simulink model "smc_rotary_pendulam"  (R2023b)
settings: Solver=VariableStepAuto  StartTime=0.0  StopTime=20  RelTol=1e-3
values from neighbouring files (symbols this model uses):
  A = double(J_subs(:,1:4))    [smc_rotary_pendulam_setup.m]
  B = double(J_subs(:,5))    [smc_rotary_pendulam_setup.m]
  D = [0,0,0,0]    [smc_rotary_pendulam_setup.m]
  K_lin = lqr(A,B,Q_1,R_1)    [smc_rotary_pendulam_setup.m]
  K_nom = -(sliding_surface*A)    [smc_rotary_pendulam_setup.m]
  sliding_surface = transpose(eig_vec(:,2))/(transpose(eig_vec(:,2))*B)    [smc_rotary_pendulam_setup.m]
undefined symbols (not defined in the file or in its folder): eig_val
libraries: simulink_extras x6
settings Model: Creator=Harishankar  LastModifiedBy=Harishankar

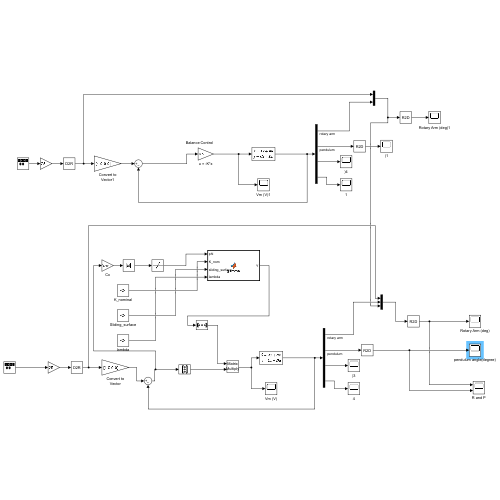
[thumbnail: Simulink's stored preview of the top-level diagram]
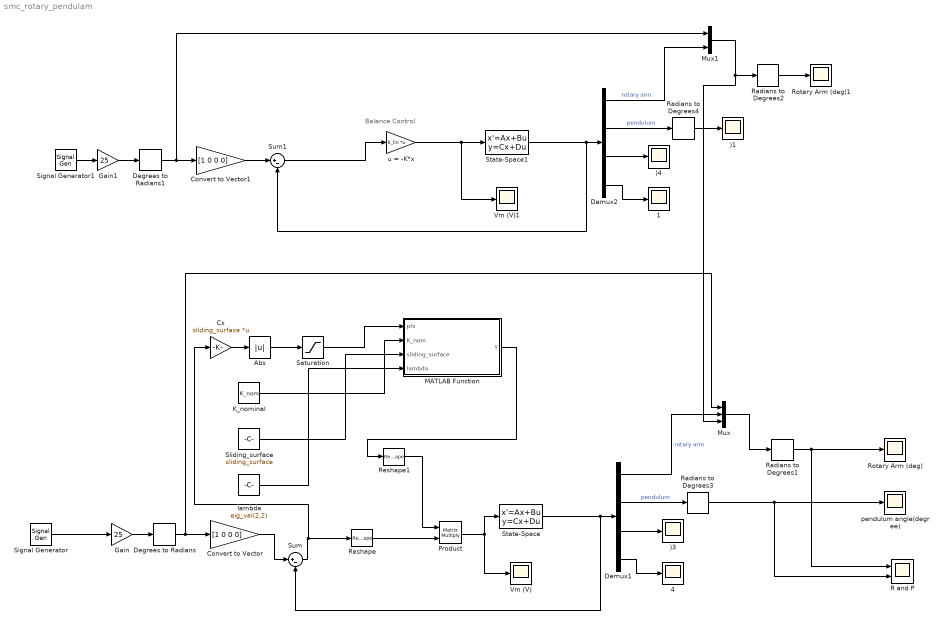
== system smc_rotary_pendulam ==
  note: Balance Control
  )1 : Scope
  )3 : Scope
  )4 : Scope
  1 : Scope
  4 : Scope
  Abs : Abs  SaturateOnIntegerOverflow=off
  Convert to Vector : Gain  Gain=[1 0 0 0]
  Convert to Vector1 : Gain  Gain=[1 0 0 0]
  Cx : Gain  Gain=sliding_surface  Multiplication=Matrix(K*u) (u vector)
  Degrees to Radians : simulink_extras/Transformations/Degrees to Radians
  Degrees to Radians1 : simulink_extras/Transformations/Degrees to Radians
  Demux1 : Demux
  Demux2 : Demux
  Gain : Gain  Gain=25
  Gain1 : Gain  Gain=25
  K_nominal : Constant  Value=K_nom
  MATLAB Function : MATLAB Function  TreatAsAtomicUnit=on
  Mux : Mux  Inputs=3
  Mux1 : Mux  Inputs=2
  Product : Product  Multiplication=Matrix(*)
  R and P : Scope  NumInputPorts=2
  Radians to Degrees{1..4} (4 alike) : simulink_extras/Transformations/Radians to Degrees
  Reshape : Reshape  OutputDimensionality=Column vector (2-D)
  Reshape1 : Reshape  OutputDimensionality=Row vector (2-D)
  Rotary Arm (deg) : Scope
  Rotary Arm (deg)1 : Scope
  Saturation : Saturate  UpperLimit=1  LowerLimit=0.35  LinearizeAsGain=off
  Signal Generator : SignalGenerator  WaveForm=square  Frequency=0.125
  Signal Generator1 : SignalGenerator  WaveForm=square  Frequency=0.125
  Sliding_surface : Constant  Value=sliding_surface
  State-Space : StateSpace  A=A  B=B  C=eye(4)  D=0*B  InitialCondition=0
  State-Space1 : StateSpace  A=A  B=B  C=eye(4)  D=0*B  InitialCondition=0
  Sum : Sum  Inputs=|+-
  Sum1 : Sum  Inputs=|+-
  Vm (V) : Scope
  Vm (V)1 : Scope
  lambda : Constant  Value=eig_val(2,2)
  pendulum angle(degree) : Scope
  u = -K*x : Gain  Gain=K_lin  Multiplication=Matrix(K*u)
  wires:
  Product/1 -> State-Space/1, Vm (V)/1
  Demux1/1 -> Mux/2  "rotary arm"
  Signal Generator/1 -> Gain/1
  Radians to Degrees3/1 -> R and P/2, pendulum angle(degree)/1
  Abs/1 -> Saturation/1
  Convert to Vector/1 -> Sum/1
  Demux1/4 -> 4/1
  Demux1/2 -> Radians to Degrees3/1  "pendulum"
  State-Space/1 -> Sum/2, Demux1/1
  Demux1/3 -> )3/1
  Saturation/1 -> MATLAB Function/1(phi)
  Sum/1 -> Reshape/1, Cx/1
  Cx/1 -> Abs/1
  Radians to Degrees1/1 -> Rotary Arm (deg)/1, R and P/1
  Gain/1 -> Degrees to Radians/1
  MATLAB Function/1(Y) -> Reshape1/1
  Mux/1 -> Radians to Degrees1/1
  Degrees to Radians/1 -> Mux/1, Convert to Vector/1
  Reshape/1 -> Product/2
  Reshape1/1 -> Product/1
  Gain1/1 -> Degrees to Radians1/1
  Demux2/3 -> )4/1
  Signal Generator1/1 -> Gain1/1
  u = -K*x/1 -> Vm (V)1/1, State-Space1/1
  Degrees to Radians1/1 -> Convert to Vector1/1, Mux1/1
  Mux1/1 -> Mux/3, Radians to Degrees2/1
  Demux2/2 -> Radians to Degrees4/1  "pendulum"
  Radians to Degrees4/1 -> )1/1
  Sum1/1 -> u = -K*x/1
  Demux2/1 -> Mux1/2  "rotary arm"
  Radians to Degrees2/1 -> Rotary Arm (deg)1/1
  Demux2/4 -> 1/1
  Convert to Vector1/1 -> Sum1/1
  State-Space1/1 -> Sum1/2, Demux2/1
  K_nominal/1 -> MATLAB Function/2(K_nom)
  Sliding_surface/1 -> MATLAB Function/3(sliding_surface)
  lambda/1 -> MATLAB Function/4(lambda)

== matlab function smc_rotary_pendulam/MATLAB Function ==
  data: phi input; Y output; K_nom input; sliding_surface input; lambda input
function Y = gamma(phi,K_nom,sliding_surface,lambda)
    % Calculate the absolute value of Cx
   
    b = 1;

    
    % Check if the absolute value is greater than or equal to b
    if phi >= b
        % If yes, use the function gtilde(absCx)
        X = lambda*sliding_surface;
    else
        % If not, assign the value b
        X= (lambda*b*sliding_surface)/phi;
    end

    Y = -1*transpose(K_nom+ X);

end
